simulink model "v3_modelo"  (R2013a)
settings: Solver=ode45  StartTime=0.0  StopTime=30  MaxStep=0.001  RelTol=1e-3
PostLoadFcn:
  | % Import the data from Excel for a lookup table
  | data_CL = xlsread('DATOS_LOOK_UP_TABLE_CL_v2','CL');
  | % Row indices for lookup table
  | breakpoints1_CL = data_CL(2:end,1)';
  | % Column indices for lookup table
  | breakpoints2_CL = data_CL(1,2:end);
  | % Output values for lookup table
  | table_data_CL = data_CL(2:end,2:end);
  | 
  | % Import the data from Excel for a lookup table
  | data_CD = xlsread('DATOS_LOOK_UP_TABLE_CL_v2','CD');
  | % Row indices for lookup table
  | breakpoints1_CD = data_CD(2:end,1)';
  | % Column indices for lookup table
  | breakpoints2_CD = data_CD(1,2:end);
  | % Output values for lookup table
  | table_data_CD = data_CD(2:end,2:end);
settings Model: Creator=Johann  LastModifiedBy=Johann

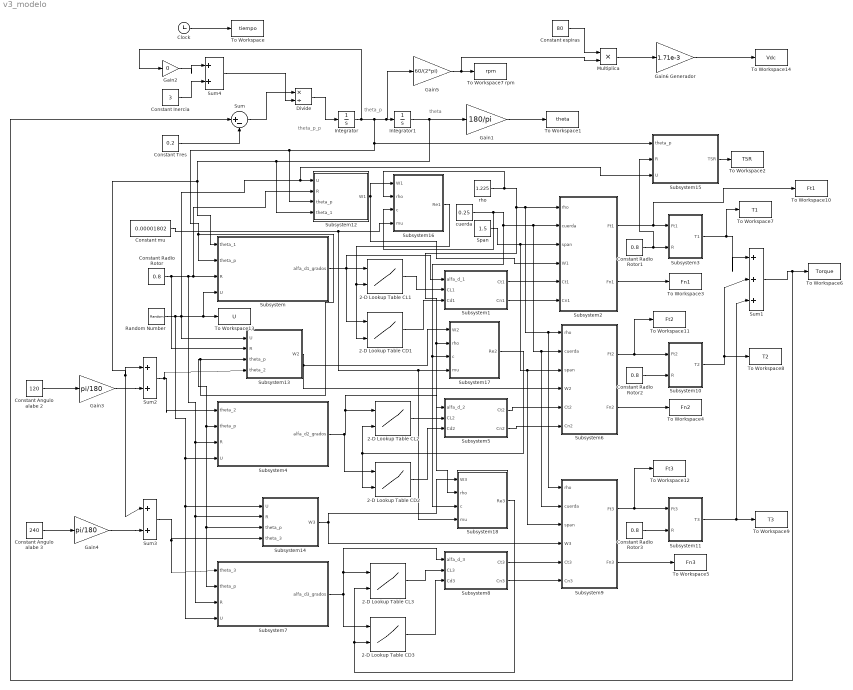
== system v3_modelo ==
  note: theta_p_p
  note: theta
  note: theta_p
  2-D Lookup Table CD1 : Lookup_n-D  BreakpointsForDimension1=breakpoints1_CD  BreakpointsForDimension2=breakpoints2_CD  Table=table_data_CD  RndMeth=Simplest  InputSameDT=on
  2-D Lookup Table CD2 : Lookup_n-D  BreakpointsForDimension1=breakpoints1_CD  BreakpointsForDimension2=breakpoints2_CD  Table=table_data_CD  RndMeth=Simplest  InputSameDT=on
  2-D Lookup Table CD3 : Lookup_n-D  BreakpointsForDimension1=breakpoints1_CD  BreakpointsForDimension2=breakpoints2_CD  Table=table_data_CD  RndMeth=Simplest  InputSameDT=on
  2-D Lookup Table CL1 : Lookup_n-D  BreakpointsForDimension1=breakpoints1_CL  BreakpointsForDimension2=breakpoints2_CL  Table=table_data_CL  RndMeth=Simplest  InputSameDT=on
  2-D Lookup Table CL2 : Lookup_n-D  BreakpointsForDimension1=breakpoints1_CL  BreakpointsForDimension2=breakpoints2_CL  Table=table_data_CL  RndMeth=Simplest  InputSameDT=on
  2-D Lookup Table CL3 : Lookup_n-D  BreakpointsForDimension1=breakpoints1_CL  BreakpointsForDimension2=breakpoints2_CL  Table=table_data_CL  RndMeth=Simplest  InputSameDT=on
  Clock : Clock
  Constant Angulo alabe 2 : Constant  Value=120
  Constant Angulo alabe 3 : Constant  Value=240
  Constant espiras : Constant  Value=80
  Constant Inercia : Constant  Value=3
  Constant Radio Rotor{,1..3} (4 alike) : Constant  Value=0.8
  Constant Tres : Constant  Value=0.2
  Constant mu : Constant  Value=0.00001802
  Divide : Product  Inputs=*/
  Gain1 : Gain  Gain=180/pi
  Gain2 : Gain  Gain=0
  Gain3 : Gain  Gain=pi/180
  Gain4 : Gain  Gain=pi/180
  Gain5 : Gain  Gain=60/(2*pi)
  Gain6 Generador : Gain  Gain=1.71e-3
  Integrator : Integrator
  Integrator1 : Integrator
  Multiplica : Product  Inputs=**
  Random Number : RandomNumber  Mean=8  Variance=4  Seed=6  SampleTime=0.1
  Span : Constant  Value=1.5
  Subsystem : Subsystem
  Subsystem1 : Subsystem
  Subsystem10 : Subsystem
  Subsystem11 : Subsystem
  Subsystem12 : Subsystem
  Subsystem13 : Subsystem
  Subsystem14 : Subsystem
  Subsystem15 : Subsystem
  Subsystem16 : Subsystem
  Subsystem17 : Subsystem
  Subsystem18 : Subsystem
  Subsystem2 : Subsystem
  Subsystem3 : Subsystem
  Subsystem4 : Subsystem
  Subsystem5 : Subsystem
  Subsystem6 : Subsystem
  Subsystem7 : Subsystem
  Subsystem8 : Subsystem
  Subsystem9 : Subsystem
  Sum : Sum  Inputs=|+-
  Sum1 : Sum  Inputs=|+++
  Sum2 : Sum  Inputs=|++
  Sum3 : Sum  Inputs=|++
  Sum4 : Sum  Inputs=|++
  To Workspace : ToWorkspace  VariableName=tiempo  SampleTime=-1
  To Workspace1 : ToWorkspace  VariableName=theta  SampleTime=-1
  To Workspace10 : ToWorkspace  VariableName=Ft1  SampleTime=-1
  To Workspace11 : ToWorkspace  VariableName=Ft2  SampleTime=-1
  To Workspace12 : ToWorkspace  VariableName=Ft3  SampleTime=-1
  To Workspace13 : ToWorkspace  VariableName=U  SampleTime=-1
  To Workspace14 : ToWorkspace  VariableName=Vdc  SampleTime=-1
  To Workspace2 : ToWorkspace  VariableName=TSR  SampleTime=-1
  To Workspace3 : ToWorkspace  VariableName=Fn1  SampleTime=-1
  To Workspace4 : ToWorkspace  VariableName=Fn2  SampleTime=-1
  To Workspace5 : ToWorkspace  VariableName=Fn3  SampleTime=-1
  To Workspace6 : ToWorkspace  VariableName=Torque  SampleTime=-1
  To Workspace7 : ToWorkspace  VariableName=T1  SampleTime=-1
  To Workspace7 rpm : ToWorkspace  VariableName=rpm  SampleTime=-1
  To Workspace8 : ToWorkspace  VariableName=T2  SampleTime=-1
  To Workspace9 : ToWorkspace  VariableName=T3  SampleTime=-1
  cuerda : Constant  Value=0.25
  rho : Constant  Value=1.225
  wires:
  Subsystem/1(alfa_d1_grados) -> 2-D Lookup Table CD1/1, Subsystem1/1(alfa_d_1), 2-D Lookup Table CL1/1
  Integrator1/1 -> Gain1/1, Subsystem12/4(theta_1), Sum2/1, Sum3/1, Subsystem/1(theta_1)
  Constant Radio Rotor/1 -> Subsystem13/2(R), Subsystem14/2(R), Subsystem7/3(R), Subsystem4/3(R), Subsystem12/2(R), Subsystem/3(R)
  Subsystem1/1(Ct1) -> Subsystem2/5(Ct1)
  Subsystem1/2(Cn1) -> Subsystem2/6(Cn1)
  cuerda/1 -> Subsystem16/3(c), Subsystem18/3(c), Subsystem17/3(c), Subsystem2/2(cuerda), Subsystem9/2(cuerda), Subsystem6/2(cuerda)
  Span/1 -> Subsystem9/3(span), Subsystem6/3(span), Subsystem2/3(span)
  Subsystem12/1(W1) -> Subsystem2/4(W1), Subsystem16/1(W1)
  Subsystem2/1(Ft1) -> To Workspace10/1, Subsystem3/1(Ft1)
  Constant Radio Rotor1/1 -> Subsystem15/2(R), Subsystem3/2(R)
  Subsystem3/1(T1) -> To Workspace7/1, Sum1/1
  Sum2/1 -> Subsystem13/4(theta_2), Subsystem4/1(theta_2)
  Subsystem4/1(alfa_d2_grados) -> 2-D Lookup Table CD2/1, Subsystem5/1(alfa_d_2), 2-D Lookup Table CL2/1
  Subsystem5/1(Ct2) -> Subsystem6/5(Ct2)
  Subsystem5/2(Cn2) -> Subsystem6/6(Cn2)
  Subsystem7/1(alfa_d3_grados) -> 2-D Lookup Table CL3/1, Subsystem8/1(alfa_d_3), 2-D Lookup Table CD3/1
  Subsystem8/1(Ct3) -> Subsystem9/5(Ct3)
  Subsystem8/2(Cn3) -> Subsystem9/6(Cn3)
  Subsystem6/1(Ft2) -> To Workspace11/1, Subsystem10/1(Ft2)
  Constant Radio Rotor2/1 -> Subsystem10/2(R)
  Subsystem10/1(T2) -> To Workspace8/1, Sum1/2
  Subsystem9/1(Ft3) -> To Workspace12/1, Subsystem11/1(Ft3)
  Constant Radio Rotor3/1 -> Subsystem11/2(R)
  Subsystem11/1(T3) -> To Workspace9/1, Sum1/3
  Sum3/1 -> Subsystem14/4(theta_3), Subsystem7/1(theta_3)
  Random Number/1 -> Subsystem14/1(U), Subsystem7/4(U), Subsystem4/4(U), Subsystem13/1(U), Subsystem15/3(U), Subsystem12/1(U), Subsystem/4(U), To Workspace13/1
  Subsystem13/1(W2) -> Subsystem6/4(W2), Subsystem17/1(W2)
  Subsystem14/1(W3) -> Subsystem9/4(W3), Subsystem18/1(W3)
  Gain1/1 -> To Workspace1/1
  Clock/1 -> To Workspace/1
  Subsystem15/1(TSR) -> To Workspace2/1
  Subsystem2/2(Fn1) -> To Workspace3/1
  Subsystem6/2(Fn2) -> To Workspace4/1
  Subsystem9/2(Fn3) -> To Workspace5/1
  Sum1/1 -> Sum/1, To Workspace6/1
  Constant mu/1 -> Subsystem18/4(mu), Subsystem17/4(mu), Subsystem16/4(mu)
  Subsystem16/1(Re1) -> 2-D Lookup Table CD1/2, 2-D Lookup Table CL1/2
  2-D Lookup Table CL1/1 -> Subsystem1/2(CL1)
  2-D Lookup Table CD1/1 -> Subsystem1/3(Cd1)
  Subsystem17/1(Re2) -> 2-D Lookup Table CL2/2, 2-D Lookup Table CD2/2
  rho/1 -> Subsystem16/2(rho), Subsystem17/2(rho), Subsystem18/2(rho), Subsystem9/1(rho), Subsystem6/1(rho), Subsystem2/1(rho)
  2-D Lookup Table CL2/1 -> Subsystem5/2(CL2)
  2-D Lookup Table CD2/1 -> Subsystem5/3(Cd2)
  Subsystem18/1(Re3) -> 2-D Lookup Table CD3/2, 2-D Lookup Table CL3/2
  2-D Lookup Table CL3/1 -> Subsystem8/2(CL3)
  2-D Lookup Table CD3/1 -> Subsystem8/3(Cd3)
  Constant Angulo alabe 2/1 -> Gain3/1
  Gain3/1 -> Sum2/2
  Constant Angulo alabe 3/1 -> Gain4/1
  Gain4/1 -> Sum3/2
  Gain5/1 -> Multiplica/2, To Workspace7 rpm/1
  Constant Tres/1 -> Sum/2
  Gain2/1 -> Sum4/1
  Constant Inercia/1 -> Sum4/2
  Sum/1 -> Divide/1
  Sum4/1 -> Divide/2
  Divide/1 -> Integrator/1
  Integrator/1 -> Gain2/1, Gain5/1, Integrator1/1, Subsystem15/1(theta_p), Subsystem12/3(theta_p), Subsystem/2(theta_p), Subsystem14/3(theta_p), Subsystem7/2(theta_p), Subsystem4/2(theta_p), Subsystem13/3(theta_p)
  Constant espiras/1 -> Multiplica/1
  Multiplica/1 -> Gain6 Generador/1
  Gain6 Generador/1 -> To Workspace14/1

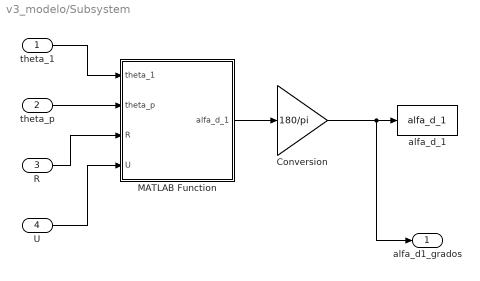
== system v3_modelo/Subsystem ==
  theta_1 : Inport
  theta_p : Inport  Port=2
  R : Inport  Port=3
  U : Inport  Port=4
  Conversion : Gain  Gain=180/pi
  MATLAB Function : MATLAB Function  TreatAsAtomicUnit=on
  alfa_d_1 : ToWorkspace  VariableName=alfa_d_1  SampleTime=-1
  alfa_d1_grados : Outport
  wires:
  MATLAB Function/1(alfa_d_1) -> Conversion/1
  Conversion/1 -> alfa_d1_grados/1, alfa_d_1/1
  theta_1/1 -> MATLAB Function/1(theta_1)
  U/1 -> MATLAB Function/4(U)
  R/1 -> MATLAB Function/3(R)
  theta_p/1 -> MATLAB Function/2(theta_p)

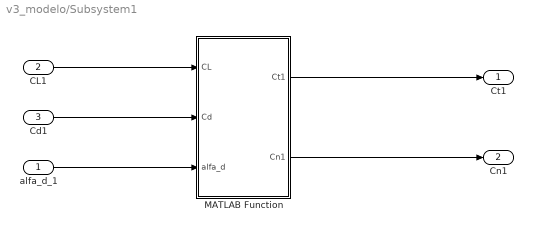
== system v3_modelo/Subsystem1 ==
  alfa_d_1 : Inport
  CL1 : Inport  Port=2
  Cd1 : Inport  Port=3
  MATLAB Function : MATLAB Function  TreatAsAtomicUnit=on
  Ct1 : Outport
  Cn1 : Outport  Port=2
  wires:
  alfa_d_1/1 -> MATLAB Function/3(alfa_d)
  Cd1/1 -> MATLAB Function/2(Cd)
  CL1/1 -> MATLAB Function/1(CL)
  MATLAB Function/1(Ct1) -> Ct1/1
  MATLAB Function/2(Cn1) -> Cn1/1

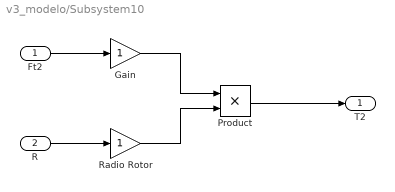
== system v3_modelo/Subsystem10 ==
  Ft2 : Inport
  R : Inport  Port=2
  Gain : Gain
  Product : Product
  Radio Rotor : Gain
  T2 : Outport
  wires:
  Ft2/1 -> Gain/1
  R/1 -> Radio Rotor/1
  Radio Rotor/1 -> Product/2
  Gain/1 -> Product/1
  Product/1 -> T2/1

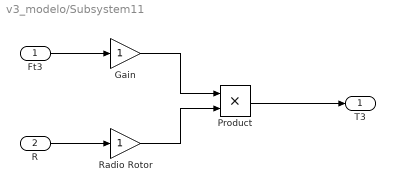
== system v3_modelo/Subsystem11 ==
  Ft3 : Inport
  R : Inport  Port=2
  Gain : Gain
  Product : Product
  Radio Rotor : Gain
  T3 : Outport
  wires:
  Ft3/1 -> Gain/1
  R/1 -> Radio Rotor/1
  Radio Rotor/1 -> Product/2
  Gain/1 -> Product/1
  Product/1 -> T3/1

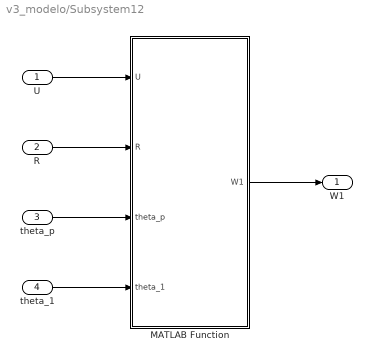
== system v3_modelo/Subsystem12 ==
  U : Inport
  R : Inport  Port=2
  theta_p : Inport  Port=3
  theta_1 : Inport  Port=4
  MATLAB Function : MATLAB Function  TreatAsAtomicUnit=on
  W1 : Outport
  wires:
  theta_1/1 -> MATLAB Function/4(theta_1)
  theta_p/1 -> MATLAB Function/3(theta_p)
  R/1 -> MATLAB Function/2(R)
  U/1 -> MATLAB Function/1(U)
  MATLAB Function/1(W1) -> W1/1

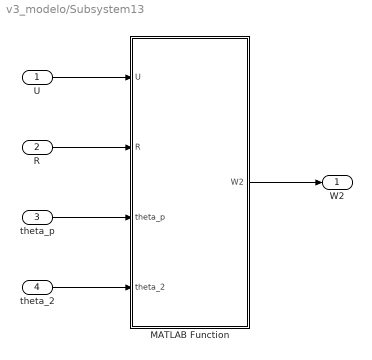
== system v3_modelo/Subsystem13 ==
  U : Inport
  R : Inport  Port=2
  theta_p : Inport  Port=3
  theta_2 : Inport  Port=4
  MATLAB Function : MATLAB Function  TreatAsAtomicUnit=on
  W2 : Outport
  wires:
  theta_2/1 -> MATLAB Function/4(theta_2)
  theta_p/1 -> MATLAB Function/3(theta_p)
  R/1 -> MATLAB Function/2(R)
  U/1 -> MATLAB Function/1(U)
  MATLAB Function/1(W2) -> W2/1

== system v3_modelo/Subsystem14 ==
  U : Inport
  R : Inport  Port=2
  theta_p : Inport  Port=3
  theta_3 : Inport  Port=4
  MATLAB Function : MATLAB Function  TreatAsAtomicUnit=on
  W3 : Outport
  wires:
  theta_3/1 -> MATLAB Function/4(theta_3)
  theta_p/1 -> MATLAB Function/3(theta_p)
  R/1 -> MATLAB Function/2(R)
  U/1 -> MATLAB Function/1(U)
  MATLAB Function/1(W3) -> W3/1

== system v3_modelo/Subsystem15 ==
  theta_p : Inport
  R : Inport  Port=2
  U : Inport  Port=3
  MATLAB Function : MATLAB Function  TreatAsAtomicUnit=on
  TSR : Outport
  wires:
  MATLAB Function/1(TSR) -> TSR/1
  theta_p/1 -> MATLAB Function/1(theta_p)
  R/1 -> MATLAB Function/2(R)
  U/1 -> MATLAB Function/3(U)

== system v3_modelo/Subsystem16 ==
  W1 : Inport
  rho : Inport  Port=2
  c : Inport  Port=3
  mu : Inport  Port=4
  MATLAB Function : MATLAB Function  TreatAsAtomicUnit=on
  Re1 : Outport
  wires:
  W1/1 -> MATLAB Function/1(W1)
  rho/1 -> MATLAB Function/2(rho)
  c/1 -> MATLAB Function/3(c)
  mu/1 -> MATLAB Function/4(mu)
  MATLAB Function/1(Re1) -> Re1/1

== system v3_modelo/Subsystem17 ==
  W2 : Inport
  rho : Inport  Port=2
  c : Inport  Port=3
  mu : Inport  Port=4
  MATLAB Function : MATLAB Function  TreatAsAtomicUnit=on
  Re2 : Outport
  wires:
  W2/1 -> MATLAB Function/1(W2)
  rho/1 -> MATLAB Function/2(rho)
  c/1 -> MATLAB Function/3(c)
  mu/1 -> MATLAB Function/4(mu)
  MATLAB Function/1(Re2) -> Re2/1

== system v3_modelo/Subsystem18 ==
  W3 : Inport
  rho : Inport  Port=2
  c : Inport  Port=3
  mu : Inport  Port=4
  MATLAB Function : MATLAB Function  TreatAsAtomicUnit=on
  Re3 : Outport
  wires:
  W3/1 -> MATLAB Function/1(W3)
  rho/1 -> MATLAB Function/2(rho)
  c/1 -> MATLAB Function/3(c)
  mu/1 -> MATLAB Function/4(mu)
  MATLAB Function/1(Re3) -> Re3/1

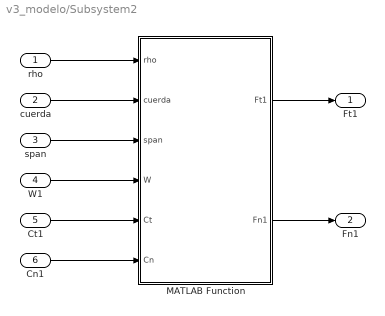
== system v3_modelo/Subsystem2 ==
  rho : Inport
  cuerda : Inport  Port=2
  span : Inport  Port=3
  W1 : Inport  Port=4
  Ct1 : Inport  Port=5
  Cn1 : Inport  Port=6
  MATLAB Function : MATLAB Function  TreatAsAtomicUnit=on
  Ft1 : Outport
  Fn1 : Outport  Port=2
  wires:
  rho/1 -> MATLAB Function/1(rho)
  cuerda/1 -> MATLAB Function/2(cuerda)
  span/1 -> MATLAB Function/3(span)
  W1/1 -> MATLAB Function/4(W)
  Ct1/1 -> MATLAB Function/5(Ct)
  Cn1/1 -> MATLAB Function/6(Cn)
  MATLAB Function/1(Ft1) -> Ft1/1
  MATLAB Function/2(Fn1) -> Fn1/1

== system v3_modelo/Subsystem3 ==
  Ft1 : Inport
  R : Inport  Port=2
  Gain : Gain
  Product : Product
  Radio Rotor : Gain
  T1 : Outport
  wires:
  Ft1/1 -> Gain/1
  R/1 -> Radio Rotor/1
  Radio Rotor/1 -> Product/2
  Gain/1 -> Product/1
  Product/1 -> T1/1

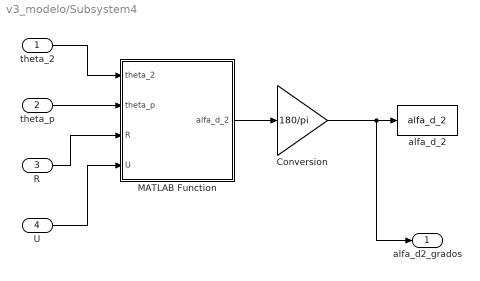
== system v3_modelo/Subsystem4 ==
  theta_2 : Inport
  theta_p : Inport  Port=2
  R : Inport  Port=3
  U : Inport  Port=4
  Conversion : Gain  Gain=180/pi
  MATLAB Function : MATLAB Function  TreatAsAtomicUnit=on
  alfa_d_2 : ToWorkspace  VariableName=alfa_d_2  SampleTime=-1
  alfa_d2_grados : Outport
  wires:
  MATLAB Function/1(alfa_d_2) -> Conversion/1
  Conversion/1 -> alfa_d2_grados/1, alfa_d_2/1
  theta_2/1 -> MATLAB Function/1(theta_2)
  U/1 -> MATLAB Function/4(U)
  R/1 -> MATLAB Function/3(R)
  theta_p/1 -> MATLAB Function/2(theta_p)

== system v3_modelo/Subsystem5 ==
  alfa_d_2 : Inport
  CL2 : Inport  Port=2
  Cd2 : Inport  Port=3
  MATLAB Function : MATLAB Function  TreatAsAtomicUnit=on
  Ct2 : Outport
  Cn2 : Outport  Port=2
  wires:
  alfa_d_2/1 -> MATLAB Function/3(alfa_d_2)
  Cd2/1 -> MATLAB Function/2(Cd2)
  CL2/1 -> MATLAB Function/1(CL2)
  MATLAB Function/1(Ct2) -> Ct2/1
  MATLAB Function/2(Cn2) -> Cn2/1

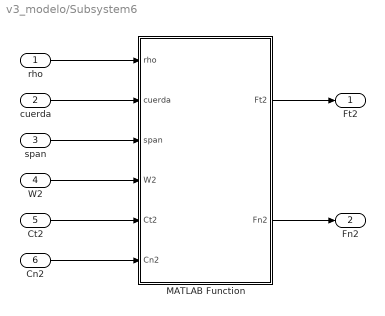
== system v3_modelo/Subsystem6 ==
  rho : Inport
  cuerda : Inport  Port=2
  span : Inport  Port=3
  W2 : Inport  Port=4
  Ct2 : Inport  Port=5
  Cn2 : Inport  Port=6
  MATLAB Function : MATLAB Function  TreatAsAtomicUnit=on
  Ft2 : Outport
  Fn2 : Outport  Port=2
  wires:
  rho/1 -> MATLAB Function/1(rho)
  cuerda/1 -> MATLAB Function/2(cuerda)
  span/1 -> MATLAB Function/3(span)
  W2/1 -> MATLAB Function/4(W2)
  Ct2/1 -> MATLAB Function/5(Ct2)
  Cn2/1 -> MATLAB Function/6(Cn2)
  MATLAB Function/1(Ft2) -> Ft2/1
  MATLAB Function/2(Fn2) -> Fn2/1

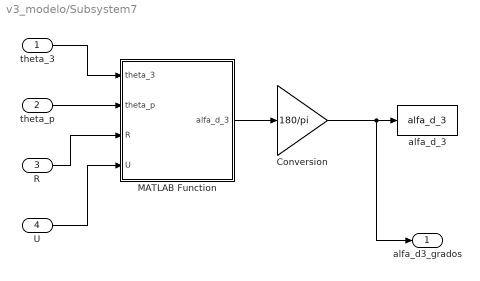
== system v3_modelo/Subsystem7 ==
  theta_3 : Inport
  theta_p : Inport  Port=2
  R : Inport  Port=3
  U : Inport  Port=4
  Conversion : Gain  Gain=180/pi
  MATLAB Function : MATLAB Function  TreatAsAtomicUnit=on
  alfa_d_3 : ToWorkspace  VariableName=alfa_d_3  SampleTime=-1
  alfa_d3_grados : Outport
  wires:
  MATLAB Function/1(alfa_d_3) -> Conversion/1
  Conversion/1 -> alfa_d3_grados/1, alfa_d_3/1
  theta_3/1 -> MATLAB Function/1(theta_3)
  U/1 -> MATLAB Function/4(U)
  R/1 -> MATLAB Function/3(R)
  theta_p/1 -> MATLAB Function/2(theta_p)

== system v3_modelo/Subsystem8 ==
  alfa_d_3 : Inport
  CL3 : Inport  Port=2
  Cd3 : Inport  Port=3
  MATLAB Function : MATLAB Function  TreatAsAtomicUnit=on
  Ct3 : Outport
  Cn3 : Outport  Port=2
  wires:
  alfa_d_3/1 -> MATLAB Function/3(alfa_d_3)
  Cd3/1 -> MATLAB Function/2(Cd3)
  CL3/1 -> MATLAB Function/1(CL3)
  MATLAB Function/1(Ct3) -> Ct3/1
  MATLAB Function/2(Cn3) -> Cn3/1

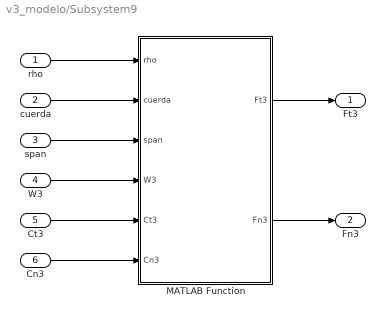
== system v3_modelo/Subsystem9 ==
  rho : Inport
  cuerda : Inport  Port=2
  span : Inport  Port=3
  W3 : Inport  Port=4
  Ct3 : Inport  Port=5
  Cn3 : Inport  Port=6
  MATLAB Function : MATLAB Function  TreatAsAtomicUnit=on
  Ft3 : Outport
  Fn3 : Outport  Port=2
  wires:
  rho/1 -> MATLAB Function/1(rho)
  cuerda/1 -> MATLAB Function/2(cuerda)
  span/1 -> MATLAB Function/3(span)
  W3/1 -> MATLAB Function/4(W3)
  Ct3/1 -> MATLAB Function/5(Ct3)
  Cn3/1 -> MATLAB Function/6(Cn3)
  MATLAB Function/1(Ft3) -> Ft3/1
  MATLAB Function/2(Fn3) -> Fn3/1

== matlab function v3_modelo/Subsystem1/MATLAB Function ==
  data: CL input; Ct1 output; Cd input; alfa_d input; Cn1 output
function [Ct1,Cn1] = conversion(CL,Cd,alfa_d)
%ENTRADAS
%CL [adimensional] Coeficiente de sustentación 
%Cd [adimensional] Coeficiente de arrastre 
%alfa_d [°] ángulo de ataque 
%**********************************************************
%SALIDAS
%Ct [adimensional] Coeficiente tangencial
%Cn [adimensional] Coeficiente normal

Ct1 = CL*sind(alfa_d)-Cd*cosd(alfa_d);

Cn1 = CL*cosd(alfa_d)+Cd*sind(alfa_d);

== matlab function v3_modelo/Subsystem/MATLAB Function ==
  data: theta_1 input; alfa_d_1 output; theta_p input; R input; U input
function alfa_d_1 = ang_ataque(theta_1,theta_p,R,U)
%ENTRADAS
%THETA_1 [rad] ángulo de azimuth para el álabe 1 
%THETA_P [rad/s] velocidad angular del rotor
%R [m] radio del rotor 
%U [m/s] velocidad de la corriente libre del viento
%**********************************************************
%SALIDA
%ALFA_D [rad]ángulo de ataque Darrieus 

%Cálculo del TSR (Tip Speed Ratio)
TSR = (theta_p*R)/U;
%Cálculo del ángulo de ataque Darrieus
alfa_d_1 = atan2(sin(theta_1),(TSR-cos(theta_1)));

== matlab function v3_modelo/Subsystem2/MATLAB Function ==
  data: rho input; Ft1 output; cuerda input; span input; W input; Ct input; Cn input; Fn1 output
function [Ft1,Fn1] = fuerzas(rho,cuerda,span,W,Ct,Cn)
%ENTRADAS
%rho [kg/m^3] Densidad del aire 
%cuerda [m] cuerda del perfil alar 
%span [m] envergadura o longitud del álabe
%W [m/s] velocidad relativa percibida por el álabe
%Ct [adimensional] Coeficiente tangencial
%Cn [adimensional] Coeficiente normal
%**********************************************************
%SALIDAS
%Ft [N] fuerza tangencial
%Fn [N] fuerza normal

Ft1 = (1/2)*(rho*cuerda*span*W^2)*Ct;
Fn1 = (1/2)*(rho*cuerda*span*W^2)*Cn;

== matlab function v3_modelo/Subsystem4/MATLAB Function ==
  data: theta_2 input; alfa_d_2 output; theta_p input; R input; U input
function alfa_d_2 = ang_ataque(theta_2,theta_p,R,U)
%ENTRADAS
%THETA_1 [rad] ángulo de azimuth para el álabe 1 
%THETA_P [rad/s] velocidad angular del rotor
%R [m] radio del rotor 
%U [m/s] velocidad de la corriente libre del viento
%**********************************************************
%SALIDA
%ALFA_D [rad]ángulo de ataque Darrieus 

%Cálculo del TSR (Tip Speed Ratio)
TSR = (theta_p*R)/U;
%Cálculo del ángulo de ataque Darrieus
alfa_d_2 = atan2(sin(theta_2),(TSR-cos(theta_2)));

== matlab function v3_modelo/Subsystem5/MATLAB Function ==
  data: CL2 input; Ct2 output; Cd2 input; alfa_d_2 input; Cn2 output
function [Ct2,Cn2] = conversion(CL2,Cd2,alfa_d_2)
%ENTRADAS
%CL [adimensional] Coeficiente de sustentación 
%Cd [adimensional] Coeficiente de arrastre 
%alfa_d [°] ángulo de ataque 
%**********************************************************
%SALIDAS
%Ct [adimensional] Coeficiente tangencial
%Cn [adimensional] Coeficiente normal

Ct2 = CL2*sind(alfa_d_2)-Cd2*cosd(alfa_d_2);

Cn2 = CL2*cosd(alfa_d_2)+Cd2*sind(alfa_d_2);

== matlab function v3_modelo/Subsystem6/MATLAB Function ==
  data: rho input; Ft2 output; cuerda input; span input; W2 input; Ct2 input; Cn2 input; Fn2 output
function [Ft2,Fn2] = fuerzas(rho,cuerda,span,W2,Ct2,Cn2)
%ENTRADAS
%rho [kg/m^3] Densidad del aire 
%cuerda [m] cuerda del perfil alar 
%span [m] envergadura o longitud del álabe
%W [m/s] velocidad relativa percibida por el álabe
%Ct [adimensional] Coeficiente tangencial
%Cn [adimensional] Coeficiente normal
%**********************************************************
%SALIDAS
%Ft [N] fuerza tangencial
%Fn [N] fuerza normal

Ft2 = (1/2)*(rho*cuerda*span*W2^2)*Ct2;
Fn2 = (1/2)*(rho*cuerda*span*W2^2)*Cn2;

== matlab function v3_modelo/Subsystem7/MATLAB Function ==
  data: theta_3 input; alfa_d_3 output; theta_p input; R input; U input
function alfa_d_3 = ang_ataque(theta_3,theta_p,R,U)
%ENTRADAS
%THETA_1 [rad] ángulo de azimuth para el álabe 1 
%THETA_P [rad/s] velocidad angular del rotor
%R [m] radio del rotor 
%U [m/s] velocidad de la corriente libre del viento
%**********************************************************
%SALIDA
%ALFA_D [rad]ángulo de ataque Darrieus 

%Cálculo del TSR (Tip Speed Ratio)
TSR = (theta_p*R)/U;
%Cálculo del ángulo de ataque Darrieus
alfa_d_3 = atan2(sin(theta_3),(TSR-cos(theta_3)));

== matlab function v3_modelo/Subsystem8/MATLAB Function ==
  data: CL3 input; Ct3 output; Cd3 input; alfa_d_3 input; Cn3 output
function [Ct3,Cn3] = conversion(CL3,Cd3,alfa_d_3)
%ENTRADAS
%CL [adimensional] Coeficiente de sustentación 
%Cd [adimensional] Coeficiente de arrastre 
%alfa_d [°] ángulo de ataque 
%**********************************************************
%SALIDAS
%Ct [adimensional] Coeficiente tangencial
%Cn [adimensional] Coeficiente normal

Ct3 = CL3*sind(alfa_d_3)-Cd3*cosd(alfa_d_3);

Cn3 = CL3*cosd(alfa_d_3)+Cd3*sind(alfa_d_3);

== matlab function v3_modelo/Subsystem9/MATLAB Function ==
  data: rho input; Ft3 output; cuerda input; span input; W3 input; Ct3 input; Cn3 input; Fn3 output
function [Ft3,Fn3] = fuerzas(rho,cuerda,span,W3,Ct3,Cn3)
%ENTRADAS
%rho [kg/m^3] Densidad del aire 
%cuerda [m] cuerda del perfil alar 
%span [m] envergadura o longitud del álabe
%W [m/s] velocidad relativa percibida por el álabe
%Ct [adimensional] Coeficiente tangencial
%Cn [adimensional] Coeficiente normal
%**********************************************************
%SALIDAS
%Ft [N] fuerza tangencial
%Fn [N] fuerza normal

Ft3 = (1/2)*(rho*cuerda*span*W3^2)*Ct3;
Fn3 = (1/2)*(rho*cuerda*span*W3^2)*Cn3;

== matlab function v3_modelo/Subsystem12/MATLAB Function ==
  data: U input; W1 output; R input; theta_p input; theta_1 input
function W1 = vel_relativa(U,R,theta_p,theta_1)
%ENTRADAS
%U [m/s] velocidad de la corriente libre del viento
%R [m] radio del rotor 
%THETA_P [rad/s] velocidad angular del rotor
%THETA_1 [rad] ángulo de azimuth para el álabe 1
%**********************************************************
%SALIDA
%W [m/s] velocidad relativa vista por el álabe 

%Cálculo del TSR (Tip Speed Ratio)
TSR = (theta_p*R)/U;
%Cálculo del ángulo de ataque Darrieus
W1 = U*sqrt((TSR^2)-2*TSR*cos(theta_1)+1);

== matlab function v3_modelo/Subsystem13/MATLAB Function ==
  data: U input; W2 output; R input; theta_p input; theta_2 input
function W2 = vel_relativa(U,R,theta_p,theta_2)
%ENTRADAS
%U [m/s] velocidad de la corriente libre del viento
%R [m] radio del rotor 
%THETA_P [rad/s] velocidad angular del rotor
%THETA_1 [rad] ángulo de azimuth para el álabe 1
%**********************************************************
%SALIDA
%W [m/s] velocidad relativa vista por el álabe 

%Cálculo del TSR (Tip Speed Ratio)
TSR = (theta_p*R)/U;
%Cálculo del ángulo de ataque Darrieus
W2 = U*sqrt((TSR^2)-2*TSR*cos(theta_2)+1);

== matlab function v3_modelo/Subsystem14/MATLAB Function ==
  data: U input; W3 output; R input; theta_p input; theta_3 input
function W3 = vel_relativa(U,R,theta_p,theta_3)
%ENTRADAS
%U [m/s] velocidad de la corriente libre del viento
%R [m] radio del rotor 
%THETA_P [rad/s] velocidad angular del rotor
%THETA_1 [rad] ángulo de azimuth para el álabe 1
%**********************************************************
%SALIDA
%W [m/s] velocidad relativa vista por el álabe 

%Cálculo del TSR (Tip Speed Ratio)
TSR = (theta_p*R)/U;
%Cálculo del ángulo de ataque Darrieus
W3 = U*sqrt((TSR^2)-2*TSR*cos(theta_3)+1);

== matlab function v3_modelo/Subsystem15/MATLAB Function ==
  data: theta_p input; TSR output; R input; U input
function TSR = TipSpeedRatio(theta_p,R,U)
%ENTRADAS
%THETA_P [rad/s] velocidad angular del rotor
%R [m] radio del rotor 
%U [m/s] velocidad de la corriente libre del viento
%**********************************************************
%SALIDA
%TSR [adimensional] razón de velocidad en la punta del álabe 

%Cálculo del TSR (Tip Speed Ratio)
TSR = (theta_p*R)/U;

== matlab function v3_modelo/Subsystem17/MATLAB Function ==
  data: W2 input; Re2 output; rho input; c input; mu input
function Re2 = fcn(W2,rho,c,mu)
%ENTRADAS
%W [m/s] velocidad relativa vista por el álabe
%RHO [kg/m^3] densidad del aire
%C [m] cuerda del perfil alar 
%MU [Pa*s] viscosidad absoluta
%**********************************************************
%SALIDA
%RE [adimensional]número de Reynolds para el álabe  
Re2 = (W2*c*rho)/mu;

== matlab function v3_modelo/Subsystem16/MATLAB Function ==
  data: W1 input; Re1 output; rho input; c input; mu input
function Re1 = fcn(W1,rho,c,mu)
%ENTRADAS
%W [m/s] velocidad relativa vista por el álabe
%RHO [kg/m^3] densidad del aire
%C [m] cuerda del perfil alar 
%MU [Pa*s] viscosidad absoluta
%**********************************************************
%SALIDA
%RE [adimensional]número de Reynolds para el álabe  
Re1 = (W1*c*rho)/mu;

== matlab function v3_modelo/Subsystem18/MATLAB Function ==
  data: W3 input; Re3 output; rho input; c input; mu input
function Re3 = fcn(W3,rho,c,mu)
%ENTRADAS
%W [m/s] velocidad relativa vista por el álabe
%RHO [kg/m^3] densidad del aire
%C [m] cuerda del perfil alar 
%MU [Pa*s] viscosidad absoluta
%**********************************************************
%SALIDA
%RE [adimensional]número de Reynolds para el álabe  
Re3 = (W3*c*rho)/mu;
